simulink subsystem "MagAngle2ReIm"  (R2023b)
settings: Solver=VariableStepAuto  StartTime=0.0  StopTime=10.0  RelTol=1e-3
settings Model: Creator=Veimar  LastModifiedBy=Veimar

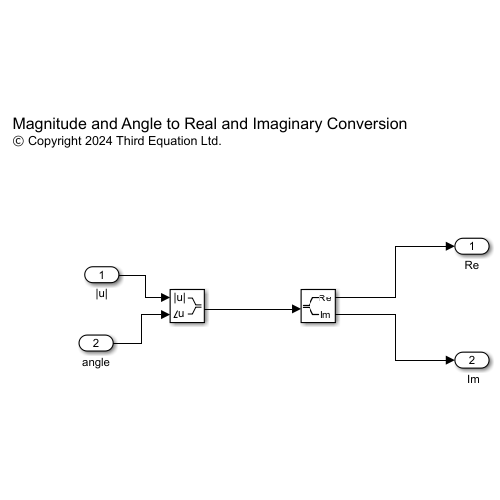
[thumbnail: Simulink's stored preview of the top-level diagram]
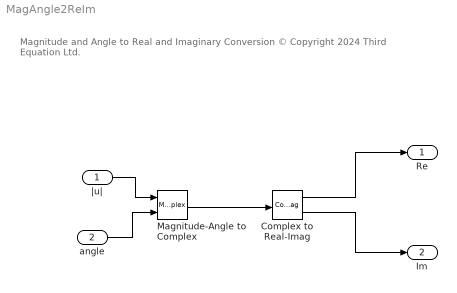
== system MagAngle2ReIm ==
  note: Magnitude and Angle to Real and Imaginary Conversion
      | © Copyright 2024 Third Equation Ltd.
  |u| : Inport
  angle : Inport  Port=2
  Complex to Real-Imag : ComplexToRealImag
  Magnitude-Angle to Complex : MagnitudeAngleToComplex
  Re : Outport
  " Im" : Outport  Port=2
  wires:
  Complex to Real-Imag/1 -> Re/1
  Magnitude-Angle to Complex/1 -> Complex to Real-Imag/1
  |u|/1 -> Magnitude-Angle to Complex/1
  angle/1 -> Magnitude-Angle to Complex/2
  Complex to Real-Imag/2 -> " Im"/1
